simulink model "FPGA_Simple_Comm"  (Simulink 7.6)
settings: Solver=FixedStepDiscrete  StartTime=0.0  StopTime=inf  FixedStep=0.01  MaxStep=1e-2  RelTol=1e-3
libraries: simulink x3
settings Model: Creator=jordan  LastModifiedBy=jordan
settings GRTTargetCC: ExtMode=on

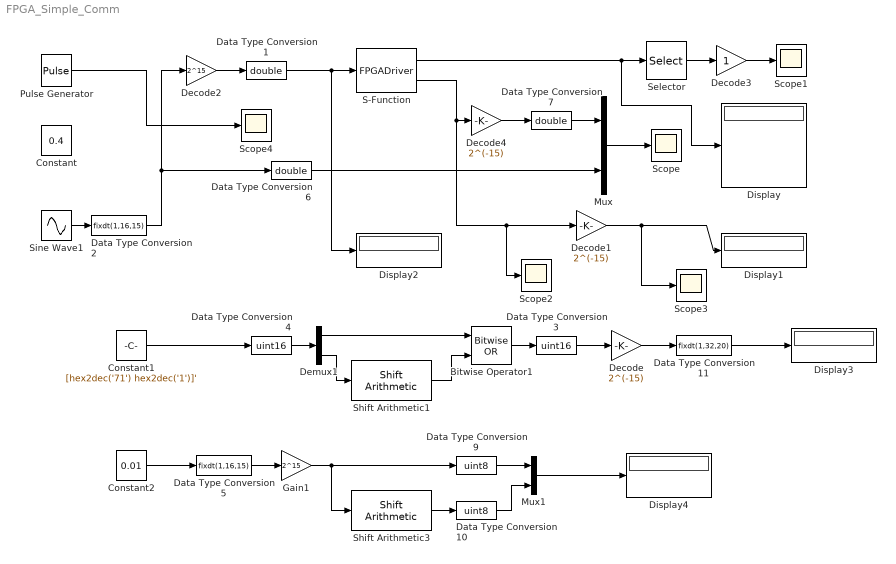
== system FPGA_Simple_Comm ==
  Bitwise Operator1 : simulink/Logic and Bit Operations/Bitwise Operator  logicop=OR  UseBitMask=off  NumInputPorts=2  BitMask=bin2dec('11011001')  BitMaskRealWorld=Stored Integer
  Constant : Constant  Value=0.4  OutDataTypeStr=double
  Constant1 : Constant  Value=[hex2dec('71') hex2dec('1')]'  OutDataTypeStr=uint8
  Constant2 : Constant  Value=0.01  OutDataTypeStr=fixdt(1,32,20)
  Data Type Conversion1 : DataTypeConversion  OutDataTypeStr=double
  Data Type Conversion10 : DataTypeConversion  OutDataTypeStr=uint8
  Data Type Conversion11 : DataTypeConversion  OutDataTypeStr=fixdt(1,32,20)
  Data Type Conversion2 : DataTypeConversion  OutDataTypeStr=fixdt(1,16,15)  SaturateOnIntegerOverflow=on
  Data Type Conversion3 : DataTypeConversion  OutDataTypeStr=uint16
  Data Type Conversion4 : DataTypeConversion  OutDataTypeStr=uint16
  Data Type Conversion5 : DataTypeConversion  OutDataTypeStr=fixdt(1,16,15)  SaturateOnIntegerOverflow=on
  Data Type Conversion6 : DataTypeConversion  OutDataTypeStr=double
  Data Type Conversion7 : DataTypeConversion  OutDataTypeStr=double
  Data Type Conversion9 : DataTypeConversion  OutDataTypeStr=uint8
  Decode : Gain  Gain=2^(-15)  OutDataTypeStr=fixdt(1,16,15)
  Decode1 : Gain  Gain=2^(-15)  OutDataTypeStr=fixdt(1,16,15)  SampleTime=0.01
  Decode2 : Gain  Gain=2^15  OutDataTypeStr=int16
  Decode3 : Gain  OutDataTypeStr=Inherit: Inherit via back propagation  SampleTime=0.01
  Decode4 : Gain  Gain=2^(-15)  OutDataTypeStr=fixdt(1,16,15)  SampleTime=0.01
  Demux1 : Demux  Outputs=2
  Display{,1..4} (5 alike) : Display
  Gain1 : Gain  Gain=2^15  OutDataTypeStr=int16  SaturateOnIntegerOverflow=on
  Mux : Mux  Inputs=2
  Mux1 : Mux  Inputs=2
  Pulse Generator : DiscretePulseGenerator  Amplitude=-1  Period=1000  PulseWidth=2  PhaseDelay=10  SampleTime=0.01
  S-Function : S-Function  FunctionName=FPGADriver  EnableBusSupport=off
  Scope{,1..4} (5 alike) : Scope
      Scope settings: TimeRange=18  YMin=-1  YMax=1
      Scope1 settings: TimeRange=14  YMin=0  YMax=275
      Scope2 settings: TimeRange=18  YMin=-1  YMax=1  SaveName=ScopeData2
      Scope3 settings: TimeRange=35  YMin=-1  YMax=1  SaveName=ScopeData3
      Scope4 settings: TimeRange=18  YMin=-1  YMax=1  SaveName=ScopeData4
  Selector : Selector  InputPortWidth=4  IndexOptions=Index vector (dialog)  Indices=2  OutputSizes=1
  Shift Arithmetic1 : simulink/Logic and Bit Operations/Shift Arithmetic  SystemSampleTime=-1  nBitShiftRight=-8  nBinPtShiftRight=0
  Shift Arithmetic3 : simulink/Logic and Bit Operations/Shift Arithmetic  SystemSampleTime=-1  nBitShiftRight=8  nBinPtShiftRight=0
  Sine Wave1 : Sin  Amplitude=0.8  Frequency=2*pi  SampleTime=0.01
  wires:
  Sine Wave1/1 -> Data Type Conversion2/1
  Mux/1 -> Scope/1
  S-Function/1 -> Selector/1, Display/1
  Selector/1 -> Decode3/1
  S-Function/2 -> Scope2/1, Decode1/1, Decode4/1
  Demux1/2 -> Shift Arithmetic1/1
  Demux1/1 -> Bitwise Operator1/1
  Shift Arithmetic1/1 -> Bitwise Operator1/2
  Bitwise Operator1/1 -> Data Type Conversion3/1
  Data Type Conversion4/1 -> Demux1/1
  Data Type Conversion3/1 -> Decode/1
  Decode/1 -> Data Type Conversion11/1
  Data Type Conversion11/1 -> Display3/1
  Constant1/1 -> Data Type Conversion4/1
  Mux1/1 -> Display4/1
  Gain1/1 -> Shift Arithmetic3/1, Data Type Conversion9/1
  Shift Arithmetic3/1 -> Data Type Conversion10/1
  Data Type Conversion9/1 -> Mux1/1
  Data Type Conversion10/1 -> Mux1/2
  Data Type Conversion5/1 -> Gain1/1
  Constant2/1 -> Data Type Conversion5/1
  Decode1/1 -> Display1/1, Scope3/1
  Decode2/1 -> Data Type Conversion1/1
  Data Type Conversion1/1 -> S-Function/1, Display2/1
  Pulse Generator/1 -> Scope4/1
  Decode3/1 -> Scope1/1
  Decode4/1 -> Data Type Conversion7/1
  Data Type Conversion2/1 -> Decode2/1, Data Type Conversion6/1
  Data Type Conversion6/1 -> Mux/2
  Data Type Conversion7/1 -> Mux/1
